simulink model "Plant"  (Simulink 7.8)
settings: Solver=FixedStepDiscrete  StartTime=0.0  StopTime=10  FixedStep=.01  RelTol=1e-3
InitFcn:
  | common
  | Busses
  | simulation_constants
  | physical_constants
values from neighbouring files (symbols this model uses):
  phi_0 = 0    [boat_constants.m]    (also in simulation_constants.m)
  wheelbase = 3.27    [boat_constants.m]
undefined symbols (not defined in the file or in its folder): DiscIntNeverNeededParam, Earth, gps_offset, gpsLatency, water_current, WGS84
libraries: aerolibtransform2 x2, uSimLib x2, simulink x1
settings Model: Creator=Bryant  LastModifiedBy=Bryant
settings DataIOCC: SignalLogging=off  DSMLogging=off
settings OptimizationCC: InlineParams=on  LifeSpan=30
settings DebuggingCC: UnderspecifiedInitializationDetection=Simplified
settings HardwareCC: ProdHWDeviceType=Generic->Unspecified (assume 32-bit Generic)  TargetIntDivRoundTo=Zero  TargetEndianess=LittleEndian  TargetHWDeviceType=Microchip->dsPIC
settings ModelReferenceCC: ModelReferenceNumInstancesAllowed=Single

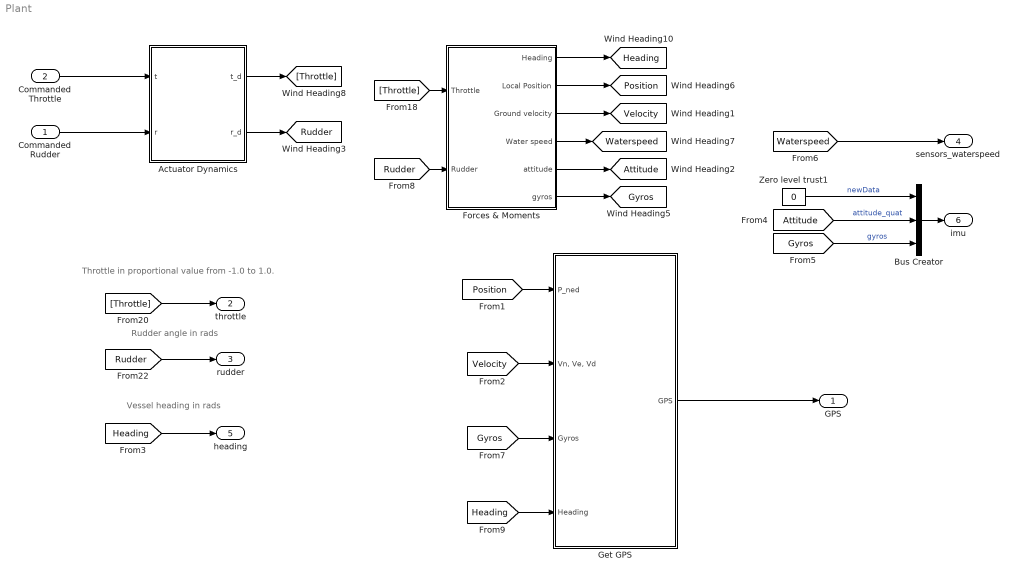
== system Plant ==
  note: Rudder angle in rads
  note: Vessel heading in rads
  note: Throttle in proportional value from -1.0 to 1.0.
  Commanded Rudder : Inport  OutDataTypeStr=single
  Commanded Throttle : Inport  Port=2  OutDataTypeStr=int16
  Actuator Dynamics : Subsystem
  Bus Creator : BusCreator  Inputs=3  OutDataTypeStr=Bus: ImuData
  Forces & Moments : Subsystem
  Get GPS : Subsystem
  Zero level trust1 : Constant  Value=0  OutDataTypeStr=boolean
  GPS : Outport  OutDataTypeStr=Bus: GpsData
  throttle : Outport  Port=2  OutDataTypeStr=double
  rudder : Outport  Port=3  OutDataTypeStr=double
  sensors_waterspeed : Outport  Port=4  OutDataTypeStr=single
  heading : Outport  Port=5  OutDataTypeStr=double
  imu : Outport  Port=6  OutDataTypeStr=Bus: ImuData
  tag scope: Attitude=global, Gyros=global, Heading=global, Position=global, Rudder=global, Velocity=global, Waterspeed=global
  wires:
  Commanded Throttle/1 -> Actuator Dynamics/1(t)
  Commanded Rudder/1 -> Actuator Dynamics/2(r)
  Actuator Dynamics/2(r_d) -> [Rudder]
  [Rudder] -> Forces & Moments/2(Rudder)
  Actuator Dynamics/1(t_d) -> [Throttle]
  [Throttle] -> Forces & Moments/1(Throttle)
  Forces & Moments/1(Heading) -> [Heading]
  [Position] -> Get GPS/1(P_ned)
  [Velocity] -> Get GPS/2("Vn, Ve, Vd")
  Get GPS/1(GPS) -> GPS/1
  [Rudder] -> rudder/1
  [Throttle] -> throttle/1
  Forces & Moments/3(Ground velocity) -> [Velocity]
  Forces & Moments/2(Local Position) -> [Position]
  [Heading] -> heading/1
  Bus Creator/1 -> imu/1
  Zero level trust1/1 -> Bus Creator/1  "newData"
  Forces & Moments/5(attitude) -> [Attitude]
  Forces & Moments/6(gyros) -> [Gyros]
  [Attitude] -> Bus Creator/2  "attitude_quat"
  [Gyros] -> Bus Creator/3  "gyros"
  Forces & Moments/4(Water speed) -> [Waterspeed]
  [Waterspeed] -> sensors_waterspeed/1
  [Gyros] -> Get GPS/3(Gyros)
  [Heading] -> Get GPS/4(Heading)

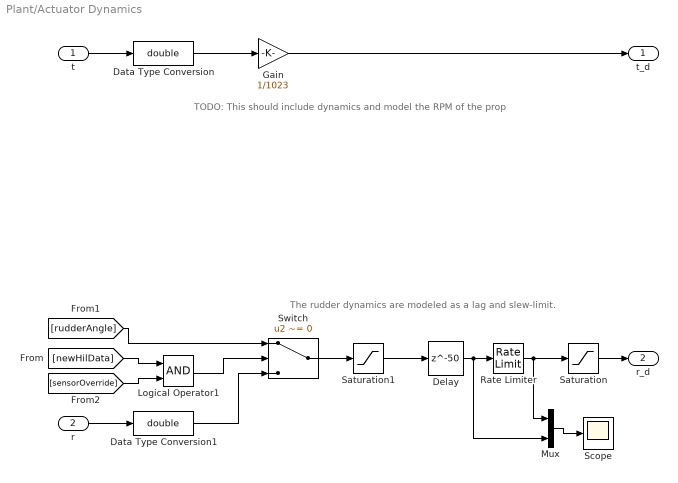
== system Plant/Actuator Dynamics ==
  note: The rudder dynamics are modeled as a lag and slew-limit.
  note: TODO: This should include dynamics and model the RPM of the prop
  t : Inport
  r : Inport  Port=2
  Data Type Conversion : DataTypeConversion  OutDataTypeStr=double  RndMeth=Simplest
  Data Type Conversion1 : DataTypeConversion  OutDataTypeStr=double  RndMeth=Simplest
  Delay : Delay  DelayLength=50
  Gain : Gain  Gain=1/1023  RndMeth=Simplest
  Logical Operator1 : Logic  AllPortsSameDT=off  OutDataTypeStr=boolean
  Mux : Mux  Inputs=2
  Rate Limiter : RateLimiter  RisingSlewLimit=0.343  FallingSlewLimit=-0.343  SampleTimeMode=inherited
  Saturation : Saturate  UpperLimit=.7854  LowerLimit=-.7854
  Saturation1 : Saturate  UpperLimit=.7854  LowerLimit=-.7854
  Scope : Scope
  Switch : Switch  Criteria=u2 ~= 0
  t_d : Outport
  r_d : Outport  Port=2
  wires:
  r/1 -> Data Type Conversion1/1
  t/1 -> Data Type Conversion/1
  [rudderAngle] -> Switch/1
  [newHilData] -> Logical Operator1/1
  [sensorOverride] -> Logical Operator1/2
  Logical Operator1/1 -> Switch/2
  Saturation/1 -> r_d/1
  Switch/1 -> Saturation1/1
  Data Type Conversion/1 -> Gain/1
  Data Type Conversion1/1 -> Switch/3
  Gain/1 -> t_d/1
  Delay/1 -> Rate Limiter/1, Mux/2
  Rate Limiter/1 -> Saturation/1, Mux/1
  Saturation1/1 -> Delay/1
  Mux/1 -> Scope/1

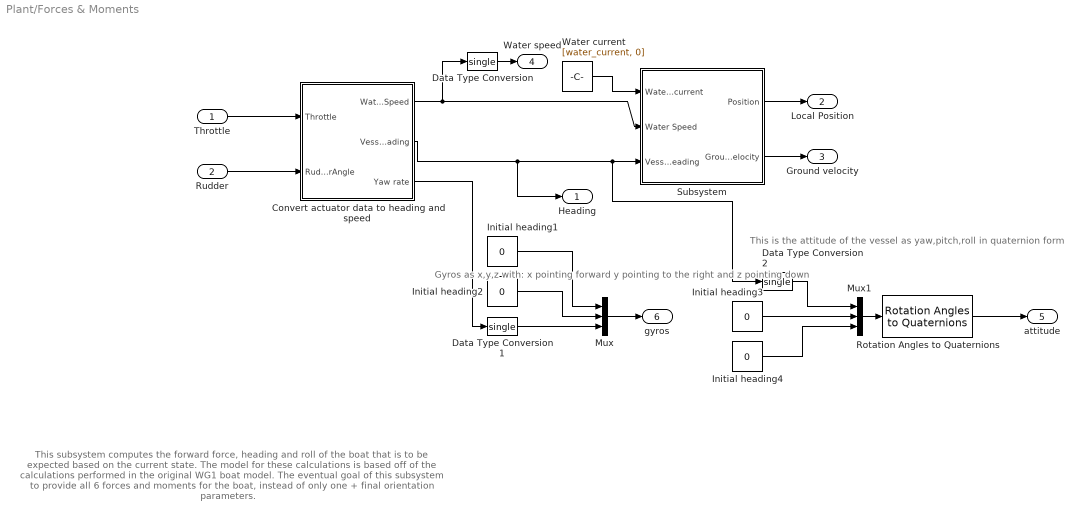
== system Plant/Forces & Moments ==
  note: This subsystem computes the forward force, heading and roll of the boat that
      | is to be expected based on the current state. The model for these calculations
      | is based off of the calculations performed in the original WG1 boat model.
      |
      | The eventual goal of this subsystem to provide all 6 forces and moments for the
      | boat, instead of only one + final orientation parameters.
  note: Gyros as x,y,z with:
      | x pointing forward
      | y pointing to the right
      | and z pointing down
  note: This is the attitude of the vessel as yaw,pitch,roll in quaternion form
  Throttle : Inport
  Rudder : Inport  Port=2
  Convert actuator data to heading and speed : Subsystem
  Data Type Conversion : DataTypeConversion  OutDataTypeStr=single  RndMeth=Simplest
  Data Type Conversion1 : DataTypeConversion  OutDataTypeStr=single  RndMeth=Simplest
  Data Type Conversion2 : DataTypeConversion  OutDataTypeStr=single  RndMeth=Simplest
  Initial heading{1..4} (4 alike) : Constant  Value=0  OutDataTypeStr=single
  Mux : Mux  Inputs=3
  Mux1 : Mux  Inputs=3
  Rotation Angles to Quaternions : aerolibtransform2/Rotation Angles to Quaternions  rotationOrder=ZYX
  Subsystem : Subsystem
  Water current : Constant  Value=[water_current, 0]
  Heading : Outport
  Local Position : Outport  Port=2
  Ground velocity : Outport  Port=3
  Water speed : Outport  Port=4
  attitude : Outport  Port=5
  gyros : Outport  Port=6
  wires:
  Throttle/1 -> Convert actuator data to heading and speed/1(Throttle)
  Rudder/1 -> Convert actuator data to heading and speed/2(RudderAngle)
  Convert actuator data to heading and speed/2(Vessel Heading) -> Heading/1, Subsystem/3(Vessel Heading), Data Type Conversion2/1
  Subsystem/1(Position) -> Local Position/1
  Convert actuator data to heading and speed/1(Water Speed) -> Subsystem/2(Water Speed), Data Type Conversion/1
  Subsystem/2(Ground Velocity) -> Ground velocity/1
  Water current/1 -> Subsystem/1(Water current)
  Data Type Conversion/1 -> Water speed/1
  Convert actuator data to heading and speed/3(Yaw rate) -> Data Type Conversion1/1
  Mux/1 -> gyros/1
  Initial heading3/1 -> Mux1/2
  Data Type Conversion2/1 -> Mux1/1
  Mux1/1 -> Rotation Angles to Quaternions/1
  Initial heading4/1 -> Mux1/3
  Rotation Angles to Quaternions/1 -> attitude/1
  Data Type Conversion1/1 -> Mux/3
  Initial heading2/1 -> Mux/2
  Initial heading1/1 -> Mux/1

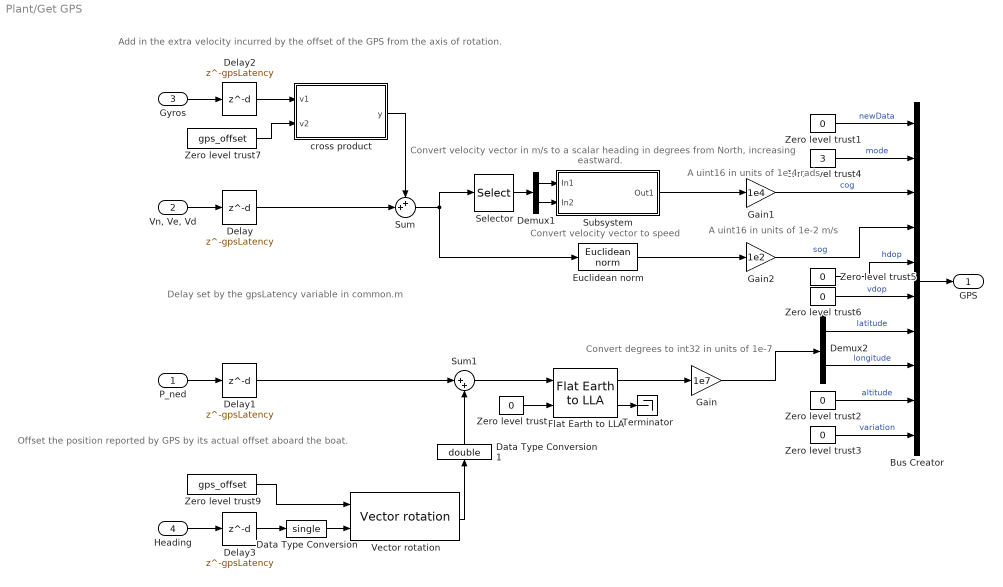
== system Plant/Get GPS ==
  note: Convert velocity vector to speed
  note: Convert velocity vector in m/s to a scalar heading
      | in degrees from North, increasing eastward.
  note: Convert degrees to
      | int32 in units of 1e-7
  note: A uint16 in units of
      | 1e-2 m/s
  note: A uint16 in units of
      | 1e-4 rads
  note: Delay set by the gpsLatency variable in common.m
  note: Add in the extra velocity incurred by the offset
      | of the GPS from the axis of rotation.
  note: Offset the position reported by GPS by its actual
      | offset aboard the boat.
  P_ned : Inport
  "Vn, Ve, Vd" : Inport  Port=2
  Gyros : Inport  Port=3
  Heading : Inport  Port=4
  Bus Creator : BusCreator  Inputs=10  OutDataTypeStr=Bus: GpsData  NonVirtualBus=on
  Data Type Conversion : DataTypeConversion  OutDataTypeStr=single  RndMeth=Simplest
  Data Type Conversion1 : DataTypeConversion  OutDataTypeStr=double  RndMeth=Simplest
  Delay{,1..3} (4 alike) : Delay  DelayLength=gpsLatency
  Demux1 : Demux  Outputs=2
  Demux2 : Demux  Outputs=2
  Euclidean norm : uSimLib/Math/Euclidean norm  SystemSampleTime=-1
  Flat Earth to LLA : aerolibtransform2/Flat Earth to LLA  units=Metric (MKS)  ptype=Earth (WGS84)  F=1/298.257223563  R=6378137  LL0=initial_LL  psi=0
  Gain : Gain  Gain=1e7  OutDataTypeStr=int32
  Gain1 : Gain  Gain=1e4  OutDataTypeStr=uint16
  Gain2 : Gain  Gain=1e2  OutDataTypeStr=uint16
  Selector : Selector  InputPortWidth=3  IndexOptions=Index vector (dialog)  Indices=[2 1]  OutputSizes=1
  Subsystem : Subsystem
  Sum : Sum  Inputs=++|
  Sum1 : Sum  Inputs=|++
  Terminator : Terminator
  Vector rotation : uSimLib/Math/Vector rotation
  Zero level trust : Constant  Value=0
  Zero level trust1 : Constant  Value=0  OutDataTypeStr=boolean
  Zero level trust2 : Constant  Value=0  OutDataTypeStr=int32
  Zero level trust3 : Constant  Value=0  OutDataTypeStr=single
  Zero level trust4 : Constant  Value=3  OutDataTypeStr=uint8
  Zero level trust5 : Constant  Value=0  OutDataTypeStr=int16
  Zero level trust6 : Constant  Value=0  OutDataTypeStr=int16
  Zero level trust7 : Constant  Value=gps_offset
  Zero level trust9 : Constant  Value=gps_offset  OutDataTypeStr=single
  cross product : MATLAB Function  TreatAsAtomicUnit=on
  GPS : Outport
  wires:
  Zero level trust/1 -> Flat Earth to LLA/2
  P_ned/1 -> Delay1/1
  Flat Earth to LLA/1 -> Gain/1
  Flat Earth to LLA/2 -> Terminator/1
  Demux2/1 -> Bus Creator/7  "latitude"
  Demux2/2 -> Bus Creator/8  "longitude"
  Euclidean norm/1 -> Gain2/1
  "Vn, Ve, Vd"/1 -> Delay/1
  Subsystem/1(Out1) -> Gain1/1
  Bus Creator/1 -> GPS/1
  Gain1/1 -> Bus Creator/3  "cog"
  Gain2/1 -> Bus Creator/4  "sog"
  Selector/1 -> Demux1/1
  Demux1/1 -> Subsystem/1(In1)
  Demux1/2 -> Subsystem/2(In2)
  Zero level trust1/1 -> Bus Creator/1  "newData"
  Gain/1 -> Demux2/1
  Zero level trust2/1 -> Bus Creator/9  "altitude"
  Zero level trust3/1 -> Bus Creator/10  "variation"
  Zero level trust4/1 -> Bus Creator/2  "mode"
  Zero level trust5/1 -> Bus Creator/5  "hdop"
  Zero level trust6/1 -> Bus Creator/6  "vdop"
  Gyros/1 -> Delay2/1
  Heading/1 -> Delay3/1
  Delay2/1 -> cross product/1(v1)
  Zero level trust7/1 -> cross product/2(v2)
  Delay/1 -> Sum/2
  Sum/1 -> Euclidean norm/1, Selector/1
  Delay1/1 -> Sum1/1
  Sum1/1 -> Flat Earth to LLA/1
  Delay3/1 -> Data Type Conversion/1
  Vector rotation/1 -> Data Type Conversion1/1
  Zero level trust9/1 -> Vector rotation/1
  Data Type Conversion/1 -> Vector rotation/2
  cross product/1(y) -> Sum/1
  Data Type Conversion1/1 -> Sum1/2

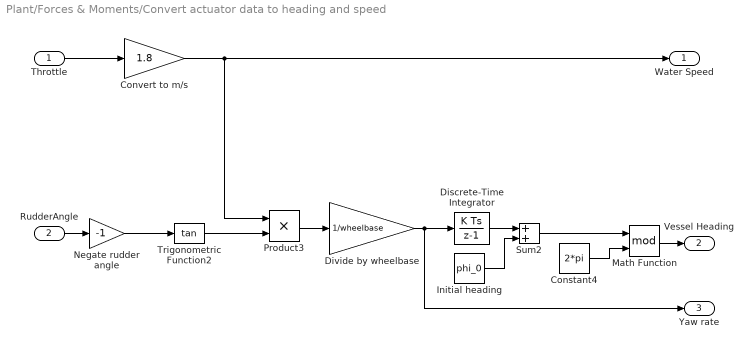
== system Plant/Forces & Moments/Convert actuator data to heading and speed ==
  Throttle : Inport
  RudderAngle : Inport  Port=2
  Constant4 : Constant  Value=2*pi
  Convert to m/s : Gain  Gain=1.8
  Discrete-Time Integrator : DiscreteIntegrator  SampleTime=.01  ICPrevOutput=DiscIntNeverNeededParam  ICPrevScaledInput=DiscIntNeverNeededParam
  Divide by wheelbase : Gain  Gain=1/wheelbase
  Initial heading : Constant  Value=phi_0
  Math Function : Math  Operator=mod  SaturateOnIntegerOverflow=on
  Negate rudder angle : Gain  Gain=-1
  Product3 : Product  RndMeth=Zero
  Sum2 : Sum  OutDataTypeStr=double
  Trigonometric Function2 : Trigonometry  Operator=tan  OutputSignalType=real
  Water Speed : Outport
  Vessel Heading : Outport  Port=2
  Yaw rate : Outport  Port=3
  wires:
  Convert to m/s/1 -> Water Speed/1, Product3/1
  Trigonometric Function2/1 -> Product3/2
  Product3/1 -> Divide by wheelbase/1
  Divide by wheelbase/1 -> Discrete-Time Integrator/1, Yaw rate/1
  Discrete-Time Integrator/1 -> Sum2/1
  Initial heading/1 -> Sum2/2
  Sum2/1 -> Math Function/1
  Negate rudder angle/1 -> Trigonometric Function2/1
  Constant4/1 -> Math Function/2
  Throttle/1 -> Convert to m/s/1
  RudderAngle/1 -> Negate rudder angle/1
  Math Function/1 -> Vessel Heading/1

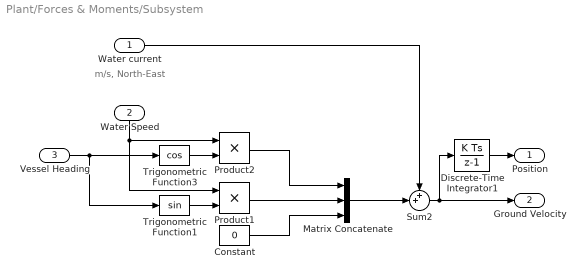
== system Plant/Forces & Moments/Subsystem ==
  note: m/s, North-East
  Water current : Inport
  Water Speed : Inport  Port=2
  Vessel Heading : Inport  Port=3
  Constant : Constant  Value=0
  Discrete-Time Integrator1 : DiscreteIntegrator  SampleTime=-1  UpperSaturationLimit=1  LowerSaturationLimit=-1  ICPrevOutput=DiscIntNeverNeededParam  ICPrevScaledInput=DiscIntNeverNeededParam
  Matrix Concatenate : Concatenate  NumInputs=3  Mode=Vector
  Product1 : Product  RndMeth=Zero
  Product2 : Product  RndMeth=Zero
  Sum2 : Sum  Inputs=++|  OutDataTypeStr=double
  Trigonometric Function1 : Trigonometry  OutputSignalType=real
  Trigonometric Function3 : Trigonometry  Operator=cos  OutputSignalType=real
  Position : Outport
  Ground Velocity : Outport  Port=2
  wires:
  Water Speed/1 -> Product2/1, Product1/1
  Trigonometric Function3/1 -> Product2/2
  Product2/1 -> Matrix Concatenate/1
  Product1/1 -> Matrix Concatenate/2
  Trigonometric Function1/1 -> Product1/2
  Constant/1 -> Matrix Concatenate/3
  Vessel Heading/1 -> Trigonometric Function3/1, Trigonometric Function1/1
  Discrete-Time Integrator1/1 -> Position/1
  Matrix Concatenate/1 -> Sum2/2
  Sum2/1 -> Discrete-Time Integrator1/1, Ground Velocity/1
  Water current/1 -> Sum2/1

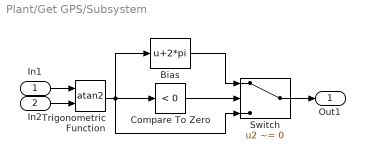
== system Plant/Get GPS/Subsystem ==
  In1 : Inport
  In2 : Inport  Port=2
  Bias : Bias  Bias=2*pi
  Compare To Zero : simulink/Logic and Bit Operations/Compare To Zero  relop=<  OutDataTypeStr=boolean
  Switch : Switch  Criteria=u2 ~= 0
  Trigonometric Function : Trigonometry  Operator=atan2
  Out1 : Outport
  wires:
  Trigonometric Function/1 -> Compare To Zero/1, Bias/1, Switch/3
  Compare To Zero/1 -> Switch/2
  Bias/1 -> Switch/1
  In1/1 -> Trigonometric Function/1
  Switch/1 -> Out1/1
  In2/1 -> Trigonometric Function/2

== matlab function Get GPS/cross product ==
  data: v1 input double size=3; y output double; v2 input double size=3
function y = cross_product(v1, v2)
%#codegen
    i = (v1(2) * v2(3) - v2(2) * v1(3));
    j = (v1(3) * v2(1) - v2(3) * v1(1));
    k = (v1(1) * v2(2) - v2(1) * v1(2));
    y = [i, j, k];
end
